simulink model "Basic_Simulation"  (R2024b)
settings: Solver=FixedStepAuto  StartTime=0.0  StopTime=inf  RelTol=1e-3
undefined symbols (not defined in the file): gray, Sim3dSensor
libraries: eeGeneralControl x4, robotcorelib x4, sim3dcameralib x2, uavsim3dlib x2, sim3dlib x1
settings Model: Creator=Sasha  LastModifiedBy=vince

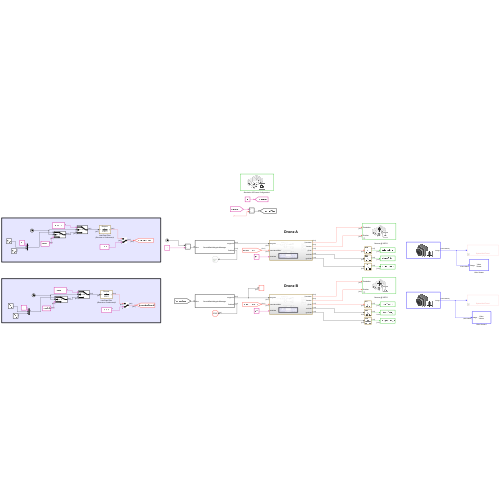
[thumbnail: Simulink's stored preview of the top-level diagram]
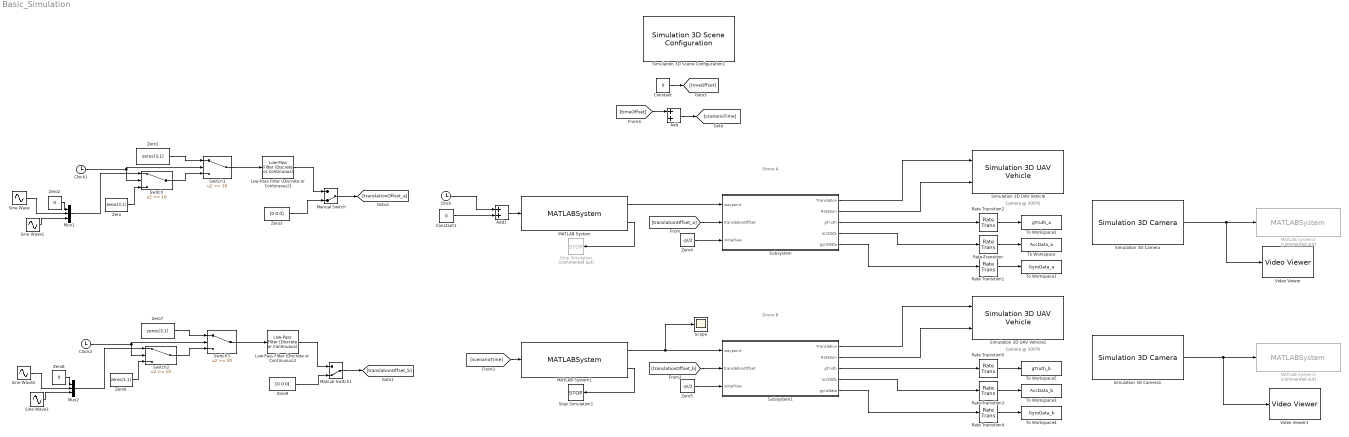
== system Basic_Simulation ==
  note: Drone A
  note: Camera @ 30FPS
  note: Camera @ 30FPS
  note: Drone B
  Add : Sum
  Add1 : Sum
  Clock : Clock
  Clock1 : Clock
  Clock2 : Clock
  Constant : Constant  Value=0
  Constant1 : Constant  Value=0
  Low-Pass Filter (Discrete or Continuous)1 : eeGeneralControl/Low-Pass Filter (Discrete or Continuous)  K=1  T=0.5  B=inf  A=-inf  init_option=Inherited from block input  x0=0  Ts=-1
  Low-Pass Filter (Discrete or Continuous)2 : eeGeneralControl/Low-Pass Filter (Discrete or Continuous)  K=1  T=0.5  B=inf  A=-inf  init_option=Inherited from block input  x0=0  Ts=-1
  MATLAB System : MATLABSystem  System=SmoothBasicWaypointManager  ScenariosDirectory=C:\Users\vince\Documents\SEN5\CollaborativeSLAM\Scenarios  ScenarioName=9a  StepTime=0.01  SimulateUsing=Interpreted execution
      mask Type: SmoothBasicWaypointManager
      mask Display:
      | disp('SmoothBasicWaypointManager');
      | port_label('input',1,'time');
      | port_label('output',1,'waypoint');
      | port_label('output',2,'finished');
  MATLAB System1 : MATLABSystem  System=SmoothBasicWaypointManager  ScenariosDirectory=C:\Users\vince\Documents\SEN5\CollaborativeSLAM\Scenarios  ScenarioName=9b  StepTime=0.01  SimulateUsing=Interpreted execution
      mask Type: SmoothBasicWaypointManager
      mask Display:
      | disp('SmoothBasicWaypointManager');
      | port_label('input',1,'time');
      | port_label('output',1,'waypoint');
      | port_label('output',2,'finished');
  MATLAB System2 : MATLABSystem  Commented=on  System=ScenarioBatchRecorder  ScenariosDirectory=C:\Users\vince\Documents\SEN5\CollaborativeSLAM\Scenarios  ScenarioName=7_a  ImageSize=[ 720, 1280 ]  BufferSize=20  EnableGrayscale=on  SimulateUsing=Interpreted execution
  MATLAB System3 : MATLABSystem  Commented=on  System=ScenarioBatchRecorder  ScenariosDirectory=C:\Users\vince\Documents\SEN5\CollaborativeSLAM\Scenarios  ScenarioName=7_b  ImageSize=[ 720, 1280 ]  BufferSize=20  EnableGrayscale=on  SimulateUsing=Interpreted execution
  Manual Switch : ManualSwitch  CurrentSetting=0
  Manual Switch1 : ManualSwitch  CurrentSetting=0
  Mux1 : Mux  Inputs=3
  Mux2 : Mux  Inputs=3
  Rate Transition{,1..5} (6 alike) : RateTransition  OutPortSampleTime=0.01
  Scope : Scope
  Simulation 3D Camera : sim3dcameralib/Simulation 3D Camera  Priority=1  sensorTag=Sim3dSensor�  sensorId=1  sensorName=Sim3dSensor�  vehTagList={'Scene Origin';'SimulinkVehicle1';'SimulinkVehicle2'}  vehTag=SimulinkVehicle1  mountLoc=Origin  offsetFlag=on  tmountOffset=[0.1, 0, 0.1]  extTmount=off  rmountOffset=[0, 0, 0]  extRmount=off  FocalLength=[1109, 1109]  OpticalCenter=[640, 360]  ImageSize=[720, 1280]  RadialDistortion=[0, 0]  TangentialDistortion=[0, 0]  SensorSkew=0  DepthOutportEnabled=off  SemanticOutportEnabled=off  TransformOutportEnabled=off  SampleTime=1/30  mountPoint=[0.1 0 0.1]  mountOrientation=[0 0 0]  aMode=3  ID=1
      settings: LibrarySourceBlock=drivingsim3d/Simulation 3D Camera
  Simulation 3D Camera1 : sim3dcameralib/Simulation 3D Camera  Priority=1  sensorTag=Sim3dSensor�  sensorId=2  sensorName=Sim3dSensor�  vehTagList={'Scene Origin';'SimulinkVehicle1';'SimulinkVehicle2'}  vehTag=SimulinkVehicle2  mountLoc=Origin  offsetFlag=on  tmountOffset=[0.1, 0, 0.1]  extTmount=off  rmountOffset=[0, 0, 0]  extRmount=off  FocalLength=[1109, 1109]  OpticalCenter=[640, 360]  ImageSize=[720, 1280]  RadialDistortion=[0, 0]  TangentialDistortion=[0, 0]  SensorSkew=0  DepthOutportEnabled=off  SemanticOutportEnabled=off  TransformOutportEnabled=off  SampleTime=1/30  mountPoint=[0.1 0 0.1]  mountOrientation=[0 0 0]  aMode=3  ID=2
      settings: LibrarySourceBlock=drivingsim3d/Simulation 3D Camera
  Simulation 3D Scene Configuration1 : sim3dlib/Simulation 3D Scene Configuration  Priority=0  ProjectFormat=Default Scenes  SceneDesc=US city block  ProjectName=C:\Program Files\MATLAB\R2024b\toolbox\shared\sim3d_projects\automotive_project_windows\UE\WindowsNoEditor\VehicleSimulation.exe  ScenePath=/Game/Maps/USCityBlock  EnableOpenDRIVE=off  vehTagList={'Custom';'Scene Origin';'SimulinkVehicle1';'SimulinkVehicle2'}  vehTag=Custom  FreeCameraInitialTranslation=[0, 0, 0]  FreeCameraDefaultInitialTranslation=[-6, 0, 2]  FreeCameraInitialRotation=[0, 0, 0]  FreeCameraDefaultInitialRotation=[0, -15, 0]  OpVisEn=off  Ts=1/100  EnableWindow=on  EnableRemoteAccess=off  EnableWeather=off  SunAzimuth=90  SunAltitude=40.0  EnableGeospatialSun=off  Latitude=0  Longitude=0  Date=2023-01-01  Time=10:30:00  GeoTimeZone=-5.0  SunDaylightSaving=off  wind=1  clouds=10  EnableVolumetricClouds=off  CloudCoverage=0  CloudAltitude=6  fog=0  rain=0  RaindropsEffect=off  SnowDensity=0  EnableGeospatial=off  UseTrueOrigin=off  OriginHeight=200  OriginLatitude=40.744652  OriginLongitude=-73.988864  MapStyle=Aerial  AdditionalAssetIDs=[]  UseAdvancedSunSky=off  SolarTime=11  TimeZone=-5  Day=21  Month=9  Year=2022  UseDaylightSavingTime=on  DSTStartDay=10  DSTStartMonth=3  DSTEndDay=3  DSTEndMonth=11  DSTSwitchHour=2  sensorTag=MainCamera2  sensorId=2  sensorName=MainCamera2  mountLoc=Origin  offsetFlag=off  tmountOffset=[0, 0, 0]  rmountOffset=[0, 0, 0]  HorizontalResolution=1280  VerticalResolution=720  HorizontalFOV=60  mountPoint=[0 0 0]  mountOrientation=[0 0 0]  aMode=4  ID=2  GeoTrigger=Inactive
      settings: LibrarySourceBlock=uavsim3dlib/Simulation 3D Scene Configuration
  Simulation 3D UAV Vehicle : uavsim3dlib/Simulation 3D UAV Vehicle  Priority=-1  Mesh=Quadrotor  MeshPath=/MathWorksUAVContent/UAVs/HexaRotorUAV/HexaRotor.HexaRotor  Color=Black  ActorName=SimulinkVehicle1  UseGlobalFrame=off  InitialTranslation=[0 0 0]  InitialRotation=[0 0 0]  InitialTranslationGlobal=[0 0 0]  InitialGeoOrigin=[0 0 0]  InitialRotationGlobal=[0 0 0]  SampleTime=1/100  ActorType=SimulinkVehicle  ID=1  aMode=4  ActorTag=SimulinkVehicle1
  Simulation 3D UAV Vehicle1 : uavsim3dlib/Simulation 3D UAV Vehicle  Priority=-1  Mesh=Quadrotor  MeshPath=/MathWorksUAVContent/UAVs/HexaRotorUAV/HexaRotor.HexaRotor  Color=Black  ActorName=SimulinkVehicle2  UseGlobalFrame=off  InitialTranslation=[0 0 0]  InitialRotation=[0 0 0]  InitialTranslationGlobal=[0 0 0]  InitialGeoOrigin=[0 0 0]  InitialRotationGlobal=[0 0 0]  SampleTime=1/100  ActorType=SimulinkVehicle  ID=2  aMode=4  ActorTag=SimulinkVehicle2
  Sine Wave : Sin  Frequency=2*pi/3  SampleTime=0
  Sine Wave1 : Sin  Frequency=2*pi/3  Phase=pi/2  SampleTime=0
  Sine Wave2 : Sin  Frequency=2*pi/3  SampleTime=0
  Sine Wave3 : Sin  Frequency=2*pi/3  Phase=pi/2  SampleTime=0
  Stop Simulation : Stop  Commented=on
  Stop Simulation1 : Stop
  Subsystem : Subsystem
  Subsystem1 : Subsystem
  Switch : Switch  Threshold=10  SaturateOnIntegerOverflow=off  InputSameDT=off
  Switch1 : Switch  Threshold=30  SaturateOnIntegerOverflow=off  InputSameDT=off
  Switch2 : Switch  Threshold=10  SaturateOnIntegerOverflow=off  InputSameDT=off
  Switch3 : Switch  Threshold=30  SaturateOnIntegerOverflow=off  InputSameDT=off
  To Workspace : ToWorkspace  VariableName=AccData_a  SaveFormat=Timeseries  SampleTime=-1
  To Workspace1 : ToWorkspace  VariableName=GyroData_a  SaveFormat=Timeseries  SampleTime=-1
  To Workspace2 : ToWorkspace  VariableName=gTruth_a  SaveFormat=Timeseries  SampleTime=-1
  To Workspace3 : ToWorkspace  VariableName=AccData_b  SaveFormat=Timeseries  SampleTime=-1
  To Workspace4 : ToWorkspace  VariableName=GyroData_b  SaveFormat=Timeseries  SampleTime=-1
  To Workspace5 : ToWorkspace  VariableName=gTruth_b  SaveFormat=Timeseries  SampleTime=-1
  Video Viewer : VideoViewer  colormapValue=gray(256)  FigPos=[2 1029 958 921]
  Video Viewer1 : VideoViewer  colormapValue=gray(256)  FigPos=[962 1029 958 921]
  Zero : Constant  Value=zeros(3,1)  VectorParams1D=off  OutDataTypeStr=Inherit: Inherit via back propagation
  Zero1 : Constant  Value=zeros(3,1)  OutDataTypeStr=Inherit: Inherit via back propagation
  Zero2 : Constant  Value=0  OutDataTypeStr=Inherit: Inherit via back propagation
  Zero3 : Constant  Value=[0 0 0]  OutDataTypeStr=Inherit: Inherit via back propagation
  Zero4 : Constant  Value=-pi/2  OutDataTypeStr=Inherit: Inherit via back propagation
  Zero5 : Constant  Value=-pi/2  OutDataTypeStr=Inherit: Inherit via back propagation
  Zero6 : Constant  Value=zeros(3,1)  VectorParams1D=off  OutDataTypeStr=Inherit: Inherit via back propagation
  Zero7 : Constant  Value=zeros(3,1)  OutDataTypeStr=Inherit: Inherit via back propagation
  Zero8 : Constant  Value=0  OutDataTypeStr=Inherit: Inherit via back propagation
  Zero9 : Constant  Value=[0 0 0]  OutDataTypeStr=Inherit: Inherit via back propagation
  wires:
  ? -> Add/2
  Constant/1 -> [timeOffset]
  MATLAB System/2 -> Stop Simulation/1
  Simulation 3D Camera/1 -> Video Viewer/1, MATLAB System2/1
  Rate Transition2/1 -> To Workspace2/1
  Switch/1 -> Switch1/3
  Zero1/1 -> Switch1/1
  Clock1/1 -> Switch/2, Switch1/2
  Sine Wave/1 -> Mux1/2
  Sine Wave1/1 -> Mux1/3
  Zero/1 -> Switch/3
  Mux1/1 -> Switch/1
  Zero2/1 -> Mux1/1
  Switch1/1 -> Low-Pass Filter (Discrete or Continuous)1/1
  Low-Pass Filter (Discrete or Continuous)1/1 -> Manual Switch/1
  Zero3/1 -> Manual Switch/2
  Manual Switch/1 -> [translationOffset_a]
  [timeOffset] -> Add/1
  Subsystem/2(Rotation) -> Simulation 3D UAV Vehicle/2
  Subsystem/1(Translation) -> Simulation 3D UAV Vehicle/1
  Subsystem/4(accData) -> Rate Transition/1
  Rate Transition/1 -> To Workspace/1
  Rate Transition1/1 -> To Workspace1/1
  Subsystem/5(gyroData) -> Rate Transition1/1
  Subsystem/3(gTruth) -> Rate Transition2/1
  MATLAB System/1 -> Subsystem/1(waypoint)
  Zero4/1 -> Subsystem/3(initialYaw)
  [translationOffset_a] -> Subsystem/2(translationOffset)
  Add/1 -> [scenarioTime]
  Clock/1 -> Add1/1
  Rate Transition3/1 -> To Workspace3/1
  Rate Transition4/1 -> To Workspace4/1
  Subsystem1/5(gyroData) -> Rate Transition4/1
  Subsystem1/2(Rotation) -> Simulation 3D UAV Vehicle1/2
  Subsystem1/1(Translation) -> Simulation 3D UAV Vehicle1/1
  Rate Transition5/1 -> To Workspace5/1
  [translationOffset_b] -> Subsystem1/2(translationOffset)
  MATLAB System1/1 -> Scope/1, Subsystem1/1(waypoint)
  Subsystem1/4(accData) -> Rate Transition3/1
  Zero5/1 -> Subsystem1/3(initialYaw)
  MATLAB System1/2 -> Stop Simulation1/1
  [scenarioTime] -> MATLAB System1/1
  Subsystem1/3(gTruth) -> Rate Transition5/1
  Simulation 3D Camera1/1 -> Video Viewer1/1, MATLAB System3/1
  Sine Wave3/1 -> Mux2/3
  Mux2/1 -> Switch2/1
  Sine Wave2/1 -> Mux2/2
  Switch3/1 -> Low-Pass Filter (Discrete or Continuous)2/1
  Zero8/1 -> Mux2/1
  Low-Pass Filter (Discrete or Continuous)2/1 -> Manual Switch1/1
  Manual Switch1/1 -> [translationOffset_b]
  Clock2/1 -> Switch2/2, Switch3/2
  Zero6/1 -> Switch2/3
  Zero9/1 -> Manual Switch1/2
  Zero7/1 -> Switch3/1
  Switch2/1 -> Switch3/3
  Add1/1 -> MATLAB System/1
  Constant1/1 -> Add1/2

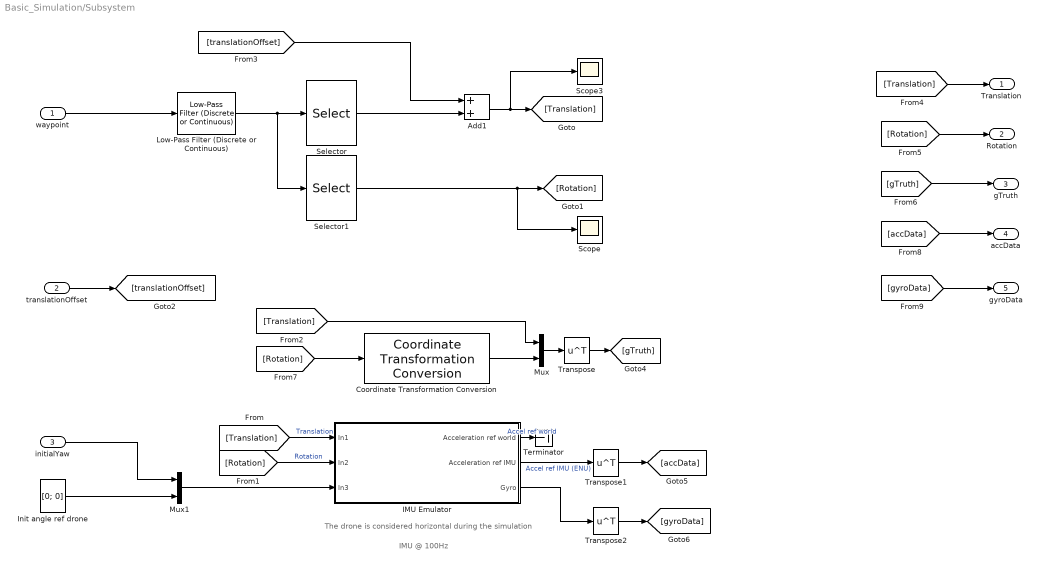
== system Basic_Simulation/Subsystem ==
  note: IMU @ 100Hz
  note: The drone is considered horizontal during the simulation
  waypoint : Inport
  translationOffset : Inport  Port=2
  initialYaw : Inport  Port=3
  Add1 : Sum
  Coordinate Transformation Conversion : robotcorelib/Coordinate Transformation Conversion  InputRepresentation=Euler Angles  InputEulerSequence=ZYX  ShowTrVecInputPort=on  OutputRepresentation=Quaternion  OutputEulerSequence=ZYX  ShowTrVecOutputPort=on  SimulateUsing=Code generation
      settings: LibrarySourceBlock=navlib/Utilities/Coordinate Transformation Conversion
  IMU Emulator : Subsystem
  Init angle ref drone : Constant  Value=[0; 0]  VectorParams1D=off
  Low-Pass Filter (Discrete or Continuous) : eeGeneralControl/Low-Pass Filter (Discrete or Continuous)  K=1  T=0.5  B=inf  A=-inf  init_option=Inherited from block input  x0=0  Ts=-1
  Mux : Mux  Inputs=2
  Mux1 : Mux  Inputs=2
  Scope : Scope
  Scope3 : Scope
  Selector : Selector  InputPortWidth=6  IndexOptions=Index vector (dialog)  Indices=[1 2 3]  OutputSizes=1
  Selector1 : Selector  InputPortWidth=6  IndexOptions=Index vector (dialog)  Indices=[4 5 6]  OutputSizes=1
  Terminator : Terminator
  Transpose : Math  Operator=transpose
  Transpose1 : Math  Operator=transpose
  Transpose2 : Math  Operator=transpose
  Translation : Outport
  Rotation : Outport  Port=2
  gTruth : Outport  Port=3
  accData : Outport  Port=4
  gyroData : Outport  Port=5
  wires:
  waypoint/1 -> Low-Pass Filter (Discrete or Continuous)/1
  Add1/1 -> Scope3/1, [Translation]
  Transpose2/1 -> [gyroData]
  Selector/1 -> Add1/2
  Init angle ref drone/1 -> Mux1/2
  Selector1/1 -> [Rotation], Scope/1
  IMU Emulator/3(Gyro) -> Transpose2/1
  Coordinate Transformation Conversion/1 -> Mux/2
  IMU Emulator/1(Acceleration ref world) -> Terminator/1  "Accel ref world"
  [translationOffset] -> Add1/1
  Mux/1 -> Transpose/1
  [Rotation] -> Coordinate Transformation Conversion/1
  Transpose1/1 -> [accData]
  Transpose/1 -> [gTruth]
  [Translation] -> Mux/1
  Low-Pass Filter (Discrete or Continuous)/1 -> Selector1/1, Selector/1
  [Rotation] -> IMU Emulator/2(In2)  "Rotation"
  [Translation] -> IMU Emulator/1(In1)  "Translation"
  IMU Emulator/2(Acceleration ref IMU) -> Transpose1/1  "Accel ref IMU (ENU)"
  [Translation] -> Translation/1
  [Rotation] -> Rotation/1
  [gTruth] -> gTruth/1
  [accData] -> accData/1
  [gyroData] -> gyroData/1
  initialYaw/1 -> Mux1/1
  Mux1/1 -> IMU Emulator/3(In3)
  translationOffset/1 -> [translationOffset]

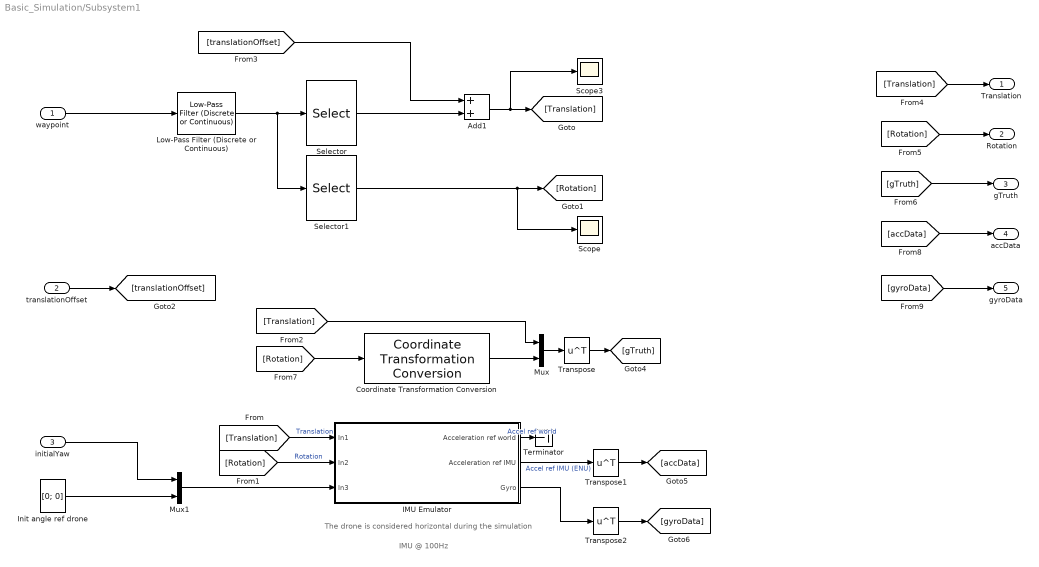
== system Basic_Simulation/Subsystem1 ==
  note: IMU @ 100Hz
  note: The drone is considered horizontal during the simulation
  waypoint : Inport
  translationOffset : Inport  Port=2
  initialYaw : Inport  Port=3
  Add1 : Sum
  Coordinate Transformation Conversion : robotcorelib/Coordinate Transformation Conversion  InputRepresentation=Euler Angles  InputEulerSequence=ZYX  ShowTrVecInputPort=on  OutputRepresentation=Quaternion  OutputEulerSequence=ZYX  ShowTrVecOutputPort=on  SimulateUsing=Code generation
  IMU Emulator : Subsystem
  Init angle ref drone : Constant  Value=[0; 0]  VectorParams1D=off
  Low-Pass Filter (Discrete or Continuous) : eeGeneralControl/Low-Pass Filter (Discrete or Continuous)  K=1  T=0.5  B=inf  A=-inf  init_option=Inherited from block input  x0=0  Ts=-1
  Mux : Mux  Inputs=2
  Mux1 : Mux  Inputs=2
  Scope : Scope
  Scope3 : Scope
  Selector : Selector  InputPortWidth=6  IndexOptions=Index vector (dialog)  Indices=[1 2 3]  OutputSizes=1
  Selector1 : Selector  InputPortWidth=6  IndexOptions=Index vector (dialog)  Indices=[4 5 6]  OutputSizes=1
  Terminator : Terminator
  Transpose : Math  Operator=transpose
  Transpose1 : Math  Operator=transpose
  Transpose2 : Math  Operator=transpose
  Translation : Outport
  Rotation : Outport  Port=2
  gTruth : Outport  Port=3
  accData : Outport  Port=4
  gyroData : Outport  Port=5
  wires:
  waypoint/1 -> Low-Pass Filter (Discrete or Continuous)/1
  Add1/1 -> Scope3/1, [Translation]
  Transpose2/1 -> [gyroData]
  Selector/1 -> Add1/2
  Init angle ref drone/1 -> Mux1/2
  Selector1/1 -> [Rotation], Scope/1
  IMU Emulator/3(Gyro) -> Transpose2/1
  Coordinate Transformation Conversion/1 -> Mux/2
  IMU Emulator/1(Acceleration ref world) -> Terminator/1  "Accel ref world"
  [translationOffset] -> Add1/1
  Mux/1 -> Transpose/1
  [Rotation] -> Coordinate Transformation Conversion/1
  Transpose1/1 -> [accData]
  Transpose/1 -> [gTruth]
  [Translation] -> Mux/1
  Low-Pass Filter (Discrete or Continuous)/1 -> Selector1/1, Selector/1
  [Rotation] -> IMU Emulator/2(In2)  "Rotation"
  [Translation] -> IMU Emulator/1(In1)  "Translation"
  IMU Emulator/2(Acceleration ref IMU) -> Transpose1/1  "Accel ref IMU (ENU)"
  [Translation] -> Translation/1
  [Rotation] -> Rotation/1
  [gTruth] -> gTruth/1
  [accData] -> accData/1
  [gyroData] -> gyroData/1
  initialYaw/1 -> Mux1/1
  Mux1/1 -> IMU Emulator/3(In3)
  translationOffset/1 -> [translationOffset]

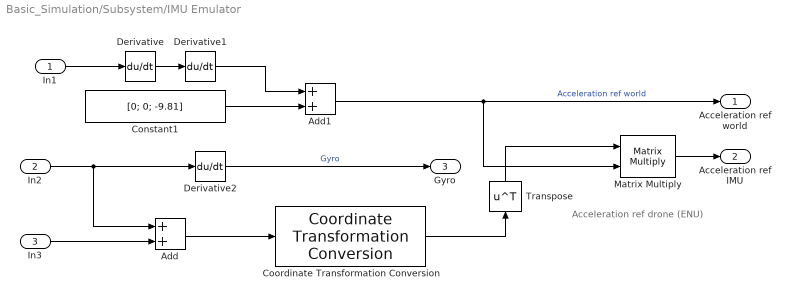
== system Basic_Simulation/Subsystem/IMU Emulator ==
  note: Acceleration ref drone (ENU)
  In1 : Inport
  In2 : Inport  Port=2
  In3 : Inport  Port=3
  Add : Sum
  Add1 : Sum
  Constant1 : Constant  Value=[0; 0; -9.81]
  Coordinate Transformation Conversion : robotcorelib/Coordinate Transformation Conversion  InputRepresentation=Euler Angles  InputEulerSequence=ZYX  ShowTrVecInputPort=on  OutputRepresentation=Rotation Matrix  OutputEulerSequence=ZYX  ShowTrVecOutputPort=on  SimulateUsing=Code generation
      settings: LibrarySourceBlock=navlib/Utilities/Coordinate Transformation Conversion
  Derivative : Derivative
  Derivative1 : Derivative
  Derivative2 : Derivative
  Matrix Multiply : Product  Multiplication=Matrix(*)
  Transpose : Math  Operator=transpose
  Acceleration ref world : Outport
  Acceleration ref IMU : Outport  Port=2
  Gyro : Outport  Port=3
  wires:
  Derivative/1 -> Derivative1/1
  Derivative2/1 -> Gyro/1  "Gyro"
  Constant1/1 -> Add1/2
  Add1/1 -> Matrix Multiply/2, Acceleration ref world/1  "Acceleration ref world"
  Derivative1/1 -> Add1/1
  In1/1 -> Derivative/1
  In2/1 -> Add/1, Derivative2/1
  In3/1 -> Add/2
  Add/1 -> Coordinate Transformation Conversion/1
  Matrix Multiply/1 -> Acceleration ref IMU/1
  Coordinate Transformation Conversion/1 -> Transpose/1
  Transpose/1 -> Matrix Multiply/1

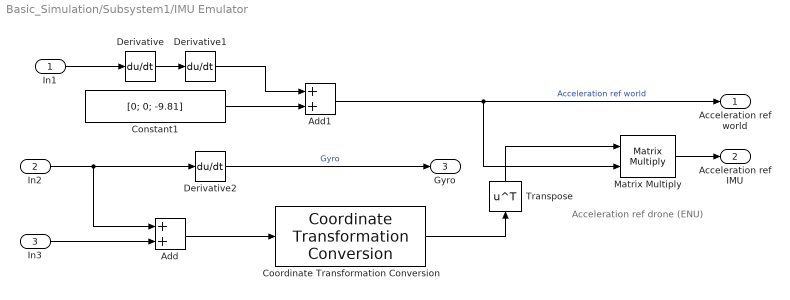
== system Basic_Simulation/Subsystem1/IMU Emulator ==
  note: Acceleration ref drone (ENU)
  In1 : Inport
  In2 : Inport  Port=2
  In3 : Inport  Port=3
  Add : Sum
  Add1 : Sum
  Constant1 : Constant  Value=[0; 0; -9.81]
  Coordinate Transformation Conversion : robotcorelib/Coordinate Transformation Conversion  InputRepresentation=Euler Angles  InputEulerSequence=ZYX  ShowTrVecInputPort=on  OutputRepresentation=Rotation Matrix  OutputEulerSequence=ZYX  ShowTrVecOutputPort=on  SimulateUsing=Code generation
  Derivative : Derivative
  Derivative1 : Derivative
  Derivative2 : Derivative
  Matrix Multiply : Product  Multiplication=Matrix(*)
  Transpose : Math  Operator=transpose
  Acceleration ref world : Outport
  Acceleration ref IMU : Outport  Port=2
  Gyro : Outport  Port=3
  wires:
  Derivative/1 -> Derivative1/1
  Derivative2/1 -> Gyro/1  "Gyro"
  Constant1/1 -> Add1/2
  Add1/1 -> Matrix Multiply/2, Acceleration ref world/1  "Acceleration ref world"
  Derivative1/1 -> Add1/1
  In1/1 -> Derivative/1
  In2/1 -> Add/1, Derivative2/1
  In3/1 -> Add/2
  Add/1 -> Coordinate Transformation Conversion/1
  Matrix Multiply/1 -> Acceleration ref IMU/1
  Coordinate Transformation Conversion/1 -> Transpose/1
  Transpose/1 -> Matrix Multiply/1
